simulink model "prova_LOG_raspi_09_22"  (R2020b)
settings: Solver=ode4  StartTime=0.0  StopTime=Inf  FixedStep=0.02  RelTol=1e-3  EnableMultiTasking=on
PostLoadFcn:
  | , if any(exist('dsrtsu_mdlpostloadfcn', 'file') == [2, 3, 6]), try dsrtsu_mdlpostloadfcn('Execute', bdroot); catch fprintf('Error in PostLoadFcn (dsrtsu_mdlpostloadfcn) for model "%s":\n %s\n', bdroot, lasterr); end, end,
InitFcn:
  | , if any(exist('rtifpga_mdlclblib', 'file') ~= 0), rtifpga_mdlclblib('Init', bdroot); end,
undefined symbols (not defined in the file or in its folder): DiscIntNeverNeededParam
libraries: simulink_extras x10, svdutilitieslib x4, raspberrypiCommlib x2, embdlinuxlib x1
Description:
  | Standard RTI1006 template.
  | Supported MATLAB version:  R2020b.
settings Model: Tag=RTI1006  DSRTSU_INTERNAL_RTI_VER=570  DSRTSU_INTERNAL_RTI_TYPE=rti1006  RTICANMMDATA=struct('GeneralSetupData',struct('modelroot','C:\SUBTEAMS_2021_2022\SOFTWARE_copia_vecchia\AUTOPILOTA\drive1\Load_hardware\Raspberry_v2_1','generalsettings',struct('filesettings',struct('destfolder',struct('Name','RTICANMM_FILES','Check',1),'buildfolder',struct('Name','.','Check',1),'AbsDestfolder',struct('Name','C:\SUBTEAMS_2021_2022\SOFTWARE_copia_vecchia\AUTOPILOTA\drive1\Load_hardware\Raspberry_v2_1\RTICANMM_FILES'),'AbsBuildfolder',struct('Name','C:\SUBTEAMS_2021_2022\SOFTWARE_copia_vecchia\AUTOPILOTA\drive1\Load_hardware\Raspberry_v2_1'))),'options',struct('addpaths',1,'rmpaths',1,'addtrcexclusion',true,'cannavigator',struct('checkmonitoring',0),'show_usrtrc',0,'use_usrtrc',0),'advanced',struct('options',ones(1,100)),'MPSetup',{{}},'RTI',struct('Type','ERT','Ver','','Date',''),'modelname','prova_LOG_raspi_09_22','block','prova_LOG_raspi_09_22'))  DSRTSU_INTERNAL_RTIFPGA=170  Creator=lapis-dspace  LastModifiedBy=lapis-dspace
settings SolverCC: PositivePriorityOrder=on
settings DataIOCC: SaveOutput=off  SignalLogging=off  DSMLogging=off  SaveTime=off  ReturnWorkspaceOutputs=off
settings OptimizationCC: EnhancedBackFolding=on  PassReuseOutputArgsAs=Individual arguments  MaxStackSize=64  OptimizeBlockOrder=speed  DifferentSizesBufferReuse=on  OptimizationCustomize=off  EfficientTunableParamExpr=on
settings DebuggingCC: ParameterTunabilityLossMsg=error  PregeneratedLibrarySubsystemCodeDiagnostic=none  ArithmeticOperatorsInVariantConditions=warning
settings HardwareCC: ProdBitPerPointer=32  ProdBitPerSizeT=32  ProdBitPerPtrDiffT=32  ProdLargestAtomicInteger=Long  ProdLargestAtomicFloat=Double  ProdWordSize=32  ProdLongLongMode=on  ProdHWDeviceType=ARM Compatible->ARM Cortex  TargetIntDivRoundTo=Zero  TargetEndianess=LittleEndian  TargetHWDeviceType=Custom Processor->Custom
settings ModelReferenceCC: ParallelModelReferenceMATLABWorkerInit=Load Top Model
settings SFSimCC: SimUseLocalCustomCode=off  MATLABDynamicMemAlloc=off  CustomCodeUndefinedFunction=UseInterfaceOnly
settings RTWCC: Description=Embedded Coder  SystemTargetFile=ert.tlc  HardwareBoard=Raspberry Pi  TLCOptions="-aInlineSetEventsForThisBaseRateFcn=TLC_FALSE -aSuppressMultiTaskScheduler=TLC_FALSE  -aRateBasedStepFcn=0"  TemplateMakefile=ert_default_tmf  GenerateReport=on  RTWUseLocalCustomCode=off  Toolchain=GNU GCC Raspberry Pi  BuildConfiguration=Faster Runs  IncludeHyperlinkInReport=on  LaunchReport=on  GenerateTraceInfo=on  GenerateTraceReport=on  GenerateTraceReportSl=on  GenerateTraceReportSf=on  GenerateTraceReportEml=on
settings CodeAppCC: ForceParamTrailComments=on  IgnoreCustomStorageClasses=off  OperatorAnnotations=on  SimulinkDataObjDesc=on  SFDataObjDesc=on  InsertBlockDesc=on
settings ERTTargetCC: MatFileLogging=on  SupportVariableSizeSignals=on
settings ConfigComp: CovMetricSettings=dswe

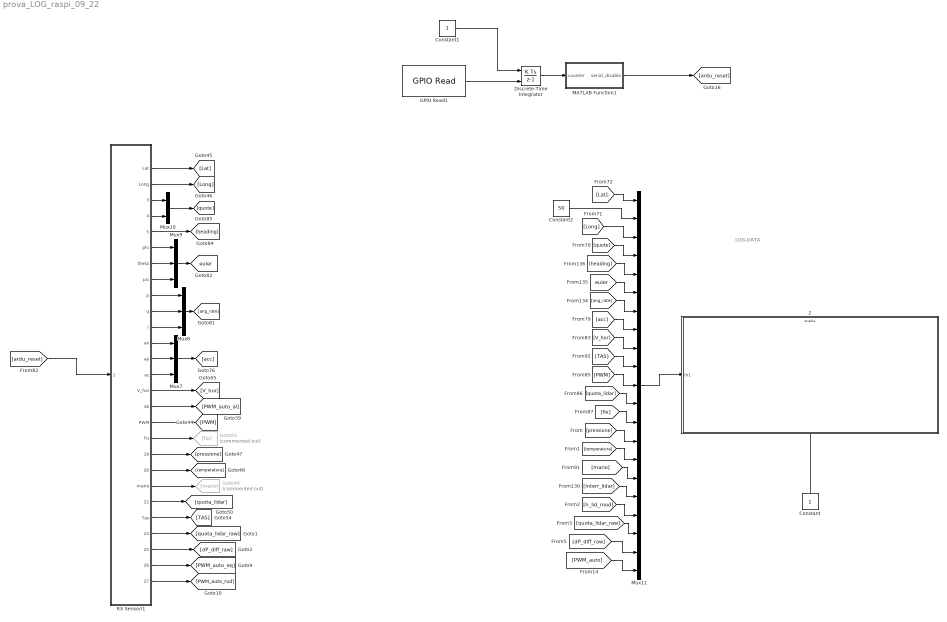
== system prova_LOG_raspi_09_22 ==
  note: LOG-DATA
  " 2" : Subsystem
  Constant : Constant
  Constant1 : Constant  SampleTime=0.02
  Constant2 : Constant  Value=50
  Discrete-Time Integrator : DiscreteIntegrator  ExternalReset=falling  SampleTime=0.02  LimitOutput=on  UpperSaturationLimit=1  LowerSaturationLimit=0  ICPrevOutput=DiscIntNeverNeededParam  ICPrevScaledInput=DiscIntNeverNeededParam
  GPIO Read1 : embdlinuxlib/GPIO Read  board=Pi 3 Model B  gpio=21  internalResistor=Off  sampleTime=0.02  direction=Input  blockPlatform=Raspberry Pi
      settings: SourceProductBaseCode=SC_BEAGLEBONE_BLUE,NVIDIA,RASPPI
  Goto49 : Goto  Commented=on  GotoTag=mario
  Goto83 : Goto  Commented=on  GotoTag=fix
  MATLAB Function1 : MATLAB Function  TreatAsAtomicUnit=on
  Mux10 : Mux  Inputs=2
  Mux11 : Mux  Inputs=21
  Mux7 : Mux  Inputs=3
  Mux8 : Mux  Inputs=3
  Mux9 : Mux  Inputs=3
  RX Sensori1 : Subsystem
  tag scope: euler=global
  wires:
  RX Sensori1/23(Tas) -> [TAS]
  RX Sensori1/10(q) -> Mux8/2
  RX Sensori1/13(ay) -> Mux7/2
  RX Sensori1/26(PWM_auto_eq) -> [PWM_auto_eq]
  RX Sensori1/4(quota_baro) -> Mux10/2
  RX Sensori1/27(PWM_auto_rud) -> [PWM_auto_rud]
  RX Sensori1/12(ax) -> Mux7/1
  RX Sensori1/14(az) -> Mux7/3
  Mux9/1 -> [euler]
  RX Sensori1/18(fix) -> Goto83/1
  RX Sensori1/25(dP_diff_raw) -> [dP_diff_raw]
  RX Sensori1/24(quota_lidar_raw) -> [quota_lidar_raw]
  RX Sensori1/15(V_hor) -> [V_hor]
  Mux8/1 -> [ang_rate]
  RX Sensori1/7(theta) -> Mux9/2
  RX Sensori1/20(temperatura) -> [temperatura]
  [ardu_reset] -> RX Sensori1/1(ardu_reset)
  RX Sensori1/5(heading) -> [heading]
  RX Sensori1/9(p) -> Mux8/1
  RX Sensori1/1(Lat) -> [Lat]
  RX Sensori1/3(quota_GPS) -> Mux10/1
  RX Sensori1/11(r) -> Mux8/3
  RX Sensori1/21(mario) -> Goto49/1
  RX Sensori1/19(pressione) -> [pressione]
  RX Sensori1/22(quota_lidar) -> [quota_lidar]
  RX Sensori1/8(psi) -> Mux9/3
  Mux10/1 -> [quote]
  RX Sensori1/16(PWM_auto_al) -> [PWM_auto_al]
  Mux7/1 -> [acc]
  RX Sensori1/2(Long) -> [Long]
  RX Sensori1/17(PWM) -> [PWM]
  RX Sensori1/6(phi) -> Mux9/1
  [acc] -> Mux11/8
  [quota_lidar_raw] -> Mux11/19
  [PWM_auto] -> Mux11/21
  [PWM] -> Mux11/11
  [dP_diff_raw] -> Mux11/20
  [h_lid_mod] -> Mux11/18
  [temperatura] -> Mux11/15
  [pressione] -> Mux11/14
  [heading] -> Mux11/5
  [Long] -> Mux11/3
  Mux11/1 -> " 2"/1(In1)
  [euler] -> Mux11/6
  [ang_rate] -> Mux11/7
  [fix] -> Mux11/13
  [Lat] -> Mux11/1
  [mario] -> Mux11/16
  [TAS] -> Mux11/10
  [quota_lidar] -> Mux11/12
  [interr_lidar] -> Mux11/17
  [quote] -> Mux11/4
  [V_hor] -> Mux11/9
  Constant/1 -> " 2"/Enable
  GPIO Read1/1 -> Discrete-Time Integrator/2
  Discrete-Time Integrator/1 -> MATLAB Function1/1(counter)
  MATLAB Function1/1(serial_disable) -> [ardu_reset]
  Constant1/1 -> Discrete-Time Integrator/1
  Constant2/1 -> Mux11/2

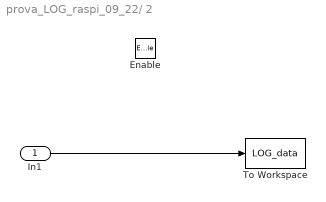
== system prova_LOG_raspi_09_22/ 2 ==
  In1 : Inport
  Enable : EnablePort
  To Workspace : ToWorkspace  VariableName=LOG_data  SaveFormat=Structure With Time  SampleTime=0.02
  wires:
  In1/1 -> To Workspace/1

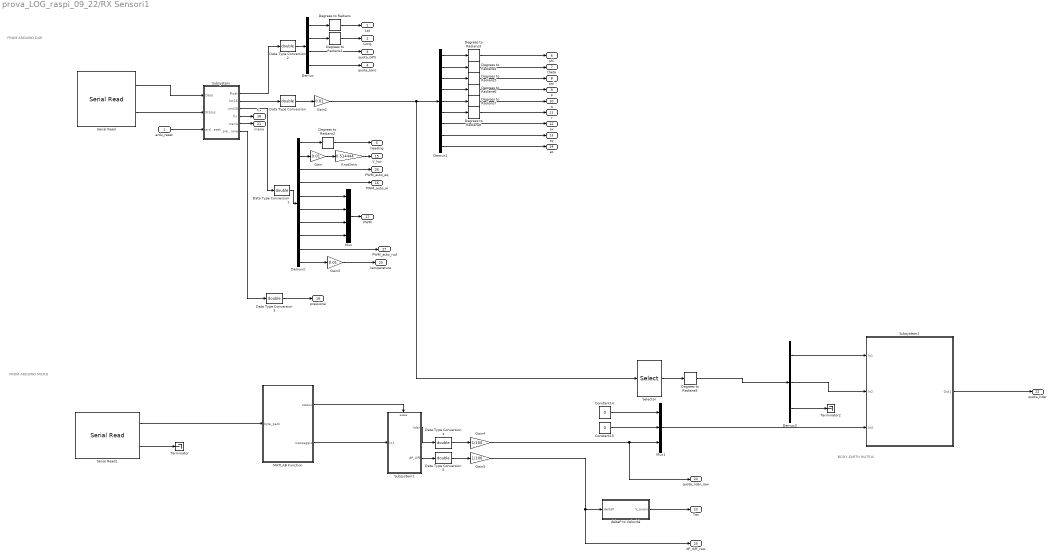
== system prova_LOG_raspi_09_22/RX Sensori1 ==
  note: FROM ARDUINO DUE
  note: FROM ARDUINO MICRO
  note: BODY-EARTH MATRIX
  ardu_reset : Inport
  Constant14 : Constant  Value=0
  Constant15 : Constant  Value=0
  Data Type Conversion{,1..5} (6 alike) : DataTypeConversion  OutDataTypeStr=double
  Degrees to Radians{,1..9} (10 alike) : simulink_extras/Transformations/Degrees to Radians
  Demux : Demux
  Demux1 : Demux  Outputs=9
  Demux2 : Demux  Outputs=10
  Demux3 : Demux  Outputs=3
  Gain : Gain  Gain=0.01
  Gain2 : Gain  Gain=0.01
  Gain3 : Gain  Gain=0.01
  Gain4 : Gain  Gain=1/100
  Gain5 : Gain  Gain=1/100
  Knot2m/s : Gain  Gain=0.514444
  MATLAB Function : MATLAB Function  TreatAsAtomicUnit=on
  Mux : Mux
  Mux1 : Mux  Inputs=3
  Selector : Selector  InputPortWidth=9  IndexOptions=Index vector (dialog)  Indices=[1:3]  OutputSizes=1
  Serial Read : raspberrypiCommlib/Serial Read  board=Pi 3 Model B+  SCIModule_=/dev/ttyACM0  Baudrate_=57600  Parity=None  StopBits_=1  HardwareFlowControl=None  ByteOrder=LittleEndian  DataLength=63  DataType=uint8  OutputStatus=on  SampleTime=0.02  blockPlatform=RaspberryPi
      settings: SourceProductBaseCode=RASPPI
  Serial Read1 : raspberrypiCommlib/Serial Read  board=Pi 3 Model B  SCIModule_=/dev/ttyACM0  Baudrate_=57600  Parity=None  StopBits_=1  HardwareFlowControl=None  ByteOrder=LittleEndian  DataLength=8  DataType=uint8  OutputStatus=on  SampleTime=0.02  blockPlatform=RaspberryPi
      settings: SourceProductBaseCode=RASPPI
  Subsystem : Subsystem
  Subsystem1 : Subsystem
  Subsystem2 : Subsystem
  Terminator : Terminator
  Terminator2 : Terminator
  deltaP to Velocità : MATLAB Function  TreatAsAtomicUnit=on
  Lat : Outport  VectorParamsAs1DForOutWhenUnconnected=off
  Long : Outport  Port=2  VectorParamsAs1DForOutWhenUnconnected=off
  quota_GPS : Outport  Port=3  VectorParamsAs1DForOutWhenUnconnected=off
  quota_baro : Outport  Port=4  VectorParamsAs1DForOutWhenUnconnected=off
  heading : Outport  Port=5  VectorParamsAs1DForOutWhenUnconnected=off
  phi : Outport  Port=6  VectorParamsAs1DForOutWhenUnconnected=off
  theta : Outport  Port=7  VectorParamsAs1DForOutWhenUnconnected=off
  psi : Outport  Port=8  VectorParamsAs1DForOutWhenUnconnected=off
  p : Outport  Port=9  VectorParamsAs1DForOutWhenUnconnected=off
  q : Outport  Port=10  VectorParamsAs1DForOutWhenUnconnected=off
  r : Outport  Port=11  VectorParamsAs1DForOutWhenUnconnected=off
  ax : Outport  Port=12  VectorParamsAs1DForOutWhenUnconnected=off
  ay : Outport  Port=13  VectorParamsAs1DForOutWhenUnconnected=off
  az : Outport  Port=14  VectorParamsAs1DForOutWhenUnconnected=off
  V_hor : Outport  Port=15  VectorParamsAs1DForOutWhenUnconnected=off
  PWM_auto_al : Outport  Port=16  VectorParamsAs1DForOutWhenUnconnected=off
  PWM : Outport  Port=17  VectorParamsAs1DForOutWhenUnconnected=off
  fix : Outport  Port=18  VectorParamsAs1DForOutWhenUnconnected=off
  pressione : Outport  Port=19  VectorParamsAs1DForOutWhenUnconnected=off
  temperatura : Outport  Port=20  VectorParamsAs1DForOutWhenUnconnected=off
  mario : Outport  Port=21  OutDataTypeStr=double  VectorParamsAs1DForOutWhenUnconnected=off
  quota_lidar : Outport  Port=22  VectorParamsAs1DForOutWhenUnconnected=off
  Tas : Outport  Port=23  VectorParamsAs1DForOutWhenUnconnected=off
  quota_lidar_raw : Outport  Port=24  VectorParamsAs1DForOutWhenUnconnected=off
  dP_diff_raw : Outport  Port=25  VectorParamsAs1DForOutWhenUnconnected=off
  PWM_auto_eq : Outport  Port=26  VectorParamsAs1DForOutWhenUnconnected=off
  PWM_auto_rud : Outport  Port=27  VectorParamsAs1DForOutWhenUnconnected=off
  wires:
  Serial Read/2 -> Subsystem/2(Status)
  Serial Read/1 -> Subsystem/1(Data)
  Subsystem/1(Float) -> Data Type Conversion2/1
  Demux/1 -> Degrees to Radians/1
  Demux/2 -> Degrees to Radians1/1
  Demux/4 -> quota_baro/1
  Subsystem/2(Int16) -> Data Type Conversion/1
  Subsystem/3(uint16) -> Data Type Conversion1/1
  Gain/1 -> Knot2m/s/1
  Demux2/3 -> PWM_auto_eq/1
  Data Type Conversion/1 -> Gain2/1
  Demux2/2 -> Gain/1
  Degrees to Radians/1 -> Lat/1
  Degrees to Radians1/1 -> Long/1
  Degrees to Radians2/1 -> heading/1
  Demux2/4 -> PWM_auto_al/1
  Demux2/7 -> Mux/3
  Demux2/8 -> Mux/4
  Data Type Conversion1/1 -> Demux2/1
  Demux2/5 -> Mux/1
  Demux2/6 -> Mux/2
  Mux/1 -> PWM/1
  Demux1/9 -> az/1
  Degrees to Radians8/1 -> r/1
  Degrees to Radians7/1 -> q/1
  Degrees to Radians6/1 -> p/1
  Degrees to Radians5/1 -> psi/1
  Degrees to Radians4/1 -> theta/1
  Degrees to Radians3/1 -> phi/1
  Demux/3 -> quota_GPS/1
  Knot2m/s/1 -> V_hor/1
  Subsystem/4(fix) -> fix/1
  Demux2/1 -> Degrees to Radians2/1
  Demux1/6 -> Degrees to Radians8/1
  Demux1/5 -> Degrees to Radians7/1
  Demux1/4 -> Degrees to Radians6/1
  Demux1/3 -> Degrees to Radians5/1
  Demux1/2 -> Degrees to Radians4/1
  Demux1/1 -> Degrees to Radians3/1
  Demux1/7 -> ax/1
  Demux1/8 -> ay/1
  Demux2/9 -> PWM_auto_rud/1
  Data Type Conversion2/1 -> Demux/1
  Gain3/1 -> temperatura/1
  Demux2/10 -> Gain3/1
  Subsystem/5(mario) -> mario/1
  Subsystem/6(pressione) -> Data Type Conversion3/1
  Data Type Conversion3/1 -> pressione/1
  ardu_reset/1 -> Subsystem/3(ardu_reset)
  MATLAB Function/2(messaggio) -> Subsystem1/1(In1)
  MATLAB Function/1(status) -> Subsystem1/Enable
  Subsystem1/1(lidar) -> Data Type Conversion4/1
  Serial Read1/1 -> MATLAB Function/1(byte_pack)
  Serial Read1/2 -> Terminator/1
  Constant15/1 -> Mux1/2
  Mux1/1 -> Subsystem2/3(In4)
  Selector/1 -> Degrees to Radians9/1
  Constant14/1 -> Mux1/1
  Degrees to Radians9/1 -> Demux3/1
  Demux3/1 -> Subsystem2/1(In1)
  Gain2/1 -> Selector/1, Demux1/1
  Data Type Conversion4/1 -> Gain4/1
  Gain4/1 -> quota_lidar_raw/1, Mux1/3
  Demux3/3 -> Terminator2/1
  Demux3/2 -> Subsystem2/2(In2)
  Subsystem2/1(Out1) -> quota_lidar/1
  Subsystem1/2(dP_diff) -> Data Type Conversion5/1
  Data Type Conversion5/1 -> Gain5/1
  deltaP to Velocità/1(V_anem) -> Tas/1
  Gain5/1 -> dP_diff_raw/1, deltaP to Velocità/1(deltaP)

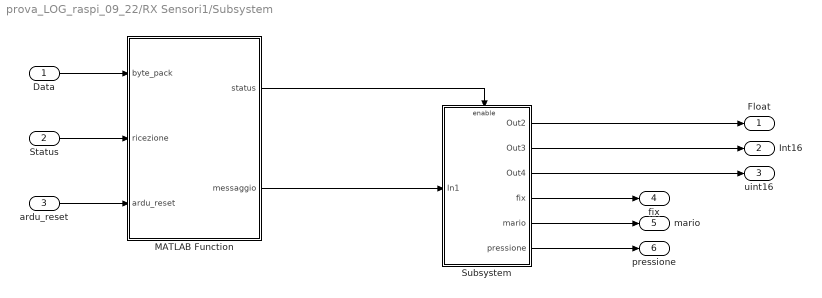
== system prova_LOG_raspi_09_22/RX Sensori1/Subsystem ==
  Data : Inport
  Status : Inport  Port=2
  ardu_reset : Inport  Port=3
  MATLAB Function : MATLAB Function  TreatAsAtomicUnit=on
  Subsystem : Subsystem
  Float : Outport  VectorParamsAs1DForOutWhenUnconnected=off
  Int16 : Outport  Port=2  VectorParamsAs1DForOutWhenUnconnected=off
  uint16 : Outport  Port=3  VectorParamsAs1DForOutWhenUnconnected=off
  fix : Outport  Port=4  VectorParamsAs1DForOutWhenUnconnected=off
  mario : Outport  Port=5  VectorParamsAs1DForOutWhenUnconnected=off
  pressione : Outport  Port=6  VectorParamsAs1DForOutWhenUnconnected=off
  wires:
  Subsystem/1(Out2) -> Float/1
  Subsystem/2(Out3) -> Int16/1
  Subsystem/3(Out4) -> uint16/1
  MATLAB Function/1(status) -> Subsystem/Enable
  MATLAB Function/2(messaggio) -> Subsystem/1(In1)
  Data/1 -> MATLAB Function/1(byte_pack)
  Status/1 -> MATLAB Function/2(ricezione)
  Subsystem/4("fix ") -> fix/1
  Subsystem/5(mario) -> mario/1
  Subsystem/6(pressione) -> pressione/1
  ardu_reset/1 -> MATLAB Function/3(ardu_reset)

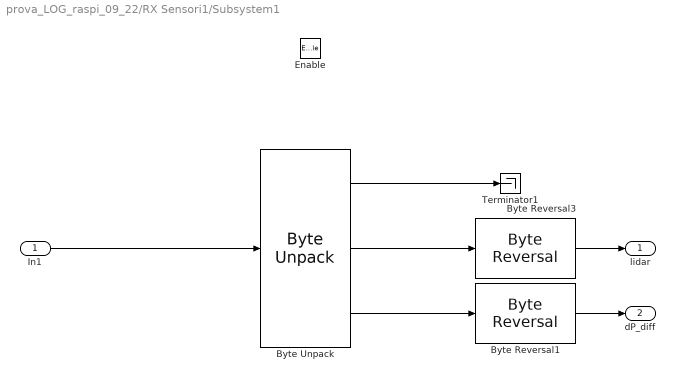
== system prova_LOG_raspi_09_22/RX Sensori1/Subsystem1 ==
  In1 : Inport
  Enable : EnablePort
  Byte Reversal1 : svdutilitieslib/Byte Reversal  numInp=1  blockPlatform=arduinoert
      settings: SourceProductBaseCode=ANDROID,ARDUINO,ML_ARDUINO,ECCORTEXA,ECCORTEXR,SC_BEAGLEBONE_BLUE,EC_FREEDOM_BOARD,EC_FRDM_K64F,INTEL_BLOCKSET,JETSONCPU,MICROBIT,NUCLEO,NVIDIA,PX4AUTOPILOTS,RASPPIIO,STMICRODIS,TIC2000,XILINX_BLOCKSET
  Byte Reversal3 : svdutilitieslib/Byte Reversal  numInp=1  blockPlatform=arduinoert
      settings: SourceProductBaseCode=ANDROID,ARDUINO,ML_ARDUINO,ECCORTEXA,ECCORTEXR,SC_BEAGLEBONE_BLUE,EC_FREEDOM_BOARD,EC_FRDM_K64F,INTEL_BLOCKSET,JETSONCPU,MICROBIT,NUCLEO,NVIDIA,PX4AUTOPILOTS,RASPPIIO,STMICRODIS,TIC2000,XILINX_BLOCKSET
  Byte Unpack : svdutilitieslib/Byte Unpack  dimensions={[2],[1],[1]}  datatypes={'uint8','uint16','int32'}  byteAlign=1  blockPlatform=arduinoert
      settings: SourceProductBaseCode=ANDROID,ARDUINO,ML_ARDUINO,ECCORTEXA,ECCORTEXR,SC_BEAGLEBONE_BLUE,EC_FREEDOM_BOARD,EC_FRDM_K64F,INTEL_BLOCKSET,JETSONCPU,MICROBIT,NUCLEO,NVIDIA,PX4AUTOPILOTS,RASPPIIO,STMICRODIS,TIC2000,XILINX_BLOCKSET
  Terminator1 : Terminator
  lidar : Outport  VectorParamsAs1DForOutWhenUnconnected=off
  dP_diff : Outport  Port=2  VectorParamsAs1DForOutWhenUnconnected=off
  wires:
  In1/1 -> Byte Unpack/1
  Byte Unpack/1 -> Terminator1/1
  Byte Unpack/2 -> Byte Reversal3/1
  Byte Reversal3/1 -> lidar/1
  Byte Unpack/3 -> Byte Reversal1/1
  Byte Reversal1/1 -> dP_diff/1

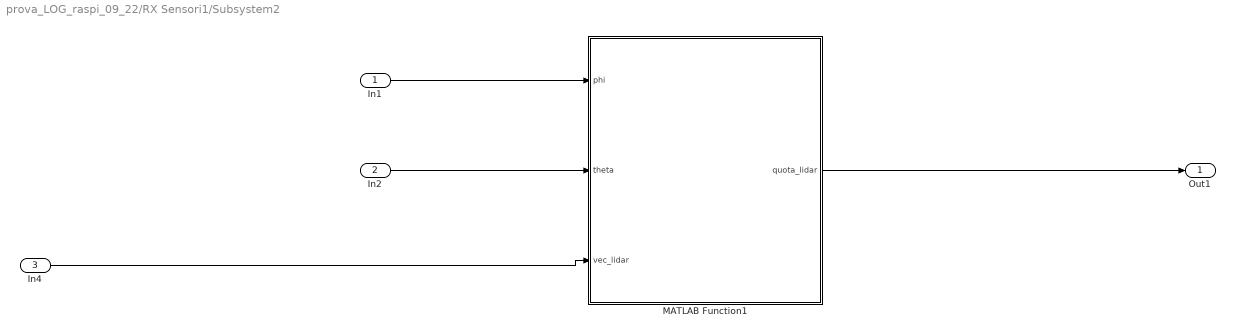
== system prova_LOG_raspi_09_22/RX Sensori1/Subsystem2 ==
  In1 : Inport
  In2 : Inport  Port=2
  In4 : Inport  Port=3
  MATLAB Function1 : MATLAB Function  TreatAsAtomicUnit=on
  Out1 : Outport  VectorParamsAs1DForOutWhenUnconnected=off
  wires:
  In4/1 -> MATLAB Function1/3(vec_lidar)
  MATLAB Function1/1(quota_lidar) -> Out1/1
  In1/1 -> MATLAB Function1/1(phi)
  In2/1 -> MATLAB Function1/2(theta)

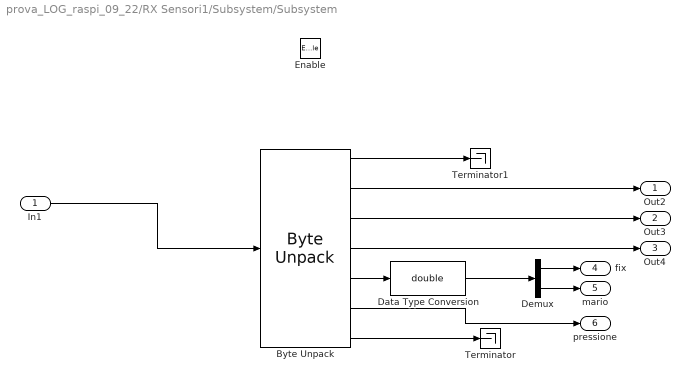
== system prova_LOG_raspi_09_22/RX Sensori1/Subsystem/Subsystem ==
  In1 : Inport
  Enable : EnablePort
  Byte Unpack : svdutilitieslib/Byte Unpack  dimensions={[2],[4],[9],[10],[2],[1],[1]}  datatypes={'uint8','single','int16','uint16','uint8','uint32','uint8'}  byteAlign=1  blockPlatform=arduinoert
      settings: SourceProductBaseCode=ANDROID,ARDUINO,ML_ARDUINO,ECCORTEXA,ECCORTEXR,SC_BEAGLEBONE_BLUE,EC_FREEDOM_BOARD,EC_FRDM_K64F,INTEL_BLOCKSET,JETSONCPU,MICROBIT,NUCLEO,NVIDIA,PX4AUTOPILOTS,RASPPIIO,STMICRODIS,TIC2000,XILINX_BLOCKSET
  Data Type Conversion : DataTypeConversion  OutDataTypeStr=double
  Demux : Demux  Outputs=2
  Terminator : Terminator
  Terminator1 : Terminator
  Out2 : Outport  VectorParamsAs1DForOutWhenUnconnected=off
  Out3 : Outport  Port=2  VectorParamsAs1DForOutWhenUnconnected=off
  Out4 : Outport  Port=3  VectorParamsAs1DForOutWhenUnconnected=off
  "fix " : Outport  Port=4  VectorParamsAs1DForOutWhenUnconnected=off
  mario : Outport  Port=5  VectorParamsAs1DForOutWhenUnconnected=off
  pressione : Outport  Port=6  VectorParamsAs1DForOutWhenUnconnected=off
  wires:
  In1/1 -> Byte Unpack/1
  Byte Unpack/1 -> Terminator1/1
  Byte Unpack/4 -> Out4/1
  Byte Unpack/3 -> Out3/1
  Byte Unpack/2 -> Out2/1
  Byte Unpack/7 -> Terminator/1
  Byte Unpack/5 -> Data Type Conversion/1
  Demux/1 -> "fix "/1
  Demux/2 -> mario/1
  Data Type Conversion/1 -> Demux/1
  Byte Unpack/6 -> pressione/1

== matlab function prova_LOG_raspi_09_22/MATLAB Function1 ==
  data: counter input; serial_disable output
function serial_disable = fcn(counter)

if counter < 1
    serial_disable = 0;
else
    serial_disable = 1;
end

== matlab function prova_LOG_raspi_09_22/RX Sensori1/deltaP to Velocità ==
  data: deltaP input; V_anem output
function V_anem = fcn(deltaP)


rho_0=1.225;
V_anem=sqrt(2*abs(deltaP)/rho_0);

== matlab function prova_LOG_raspi_09_22/RX Sensori1/MATLAB Function ==
  data: byte_pack input; status output; messaggio output
function [status,messaggio]  = LETTURA_Arduino_mex(byte_pack)



status = false;                                        %ho aggiunto questo
messaggio = uint8(zeros(1,8)) ;
M = uint8(length(byte_pack)) ;

 





    for i = 1 : M-1  
        if ( byte_pack(i) == 254 &&  byte_pack(i + 1) == 255 )                  % mi conviene mandare un secondo byte all'inizio cosi non devo cambiare nulla
            messaggio(1:end) = byte_pack(i:i+7) ;
            status = true ; 
            break
        end
    end   % lho messo qua

== matlab function prova_LOG_raspi_09_22/RX Sensori1/Subsystem/MATLAB Function ==
  data: byte_pack input; status output; messaggio output; ricezione input; ardu_reset input
function [status,messaggio]  = LETTURA_Arduino_mex(byte_pack,ricezione,ardu_reset)

persistent message counter start_found

status = false;                                        %ho aggiunto questo
messaggio = uint8(zeros(1,63)) ;
M = uint8(length(byte_pack)) ;
entrata = true ;

if isempty(start_found) 
     start_found = false ;
end 
if isempty (counter) 
    counter = uint8(0) ;
end 
if isempty(message)
     message = uint8(zeros(1,63)) ;
end

if ((ricezione ~= 0) || (ardu_reset == 0))
    start_found = false ;
    message = uint8(zeros(1,63)) ;
    counter = uint8(0)  ;
    entrata = false ;
end

if (start_found == 0 && entrata == true )
    for i = 1 : M-1  
        if ( byte_pack(i) == 62 &&  byte_pack(i + 1) == 255 )                  % mi conviene mandare un secondo byte all'inizio cosi non devo cambiare nulla
            message(1:M - (i-1)) = byte_pack(i:end) ;
            counter = M - (i-1) ; 
            start_found = true ;
            break
        end
    end   % lho messo qua
        if counter == M 
            messaggio = message ;
            message = uint8(zeros(1,63)) ;
            status = true ;
            start_found = false ;
            counter = uint8(0) ;
        end
     %end
    
    
elseif start_found == 1 

        message(counter + 1 : end) = byte_pack(1:M - counter) ;
        status = true;       %ho aggiunto questo
        messaggio = message ;
        counter = M - counter ;
        message = uint8(zeros(1,63)) ;
        
            for i = counter : M-1  
        if ( byte_pack(i) == 62 &&  byte_pack(i + 1) == 255 )                  % mi conviene mandare un secondo byte all'inizio cosi non devo cambiare nulla
            message(1:M - (i-1)) = byte_pack(i:end) ;
            counter = M - (i-1) ; 
            start_found = true ;
            break
        else 
            start_found = false ;
            counter = uint8(0);
        end 
            end
        
     %   message (1 : M-counter ) = byte_pack(counter + 1:end) ;
     %   counter = M - counter ;

end

== matlab function prova_LOG_raspi_09_22/RX Sensori1/Subsystem2/MATLAB Function1 ==
  data: phi input; quota_lidar output; theta input; vec_lidar input
function quota_lidar = fcn(phi,theta,vec_lidar)

vec_quota = [0; 0; 0];


LBE = [cos(theta)           sin(phi)*sin(theta)       cos(phi)*sin(theta);
       0                       cos(phi)                  -sin(phi);
       -sin(theta)          cos(theta)*sin(phi)       cos(phi)*cos(theta)];
       

vec_quota = LBE*vec_lidar;   % componenti della quota lidar in assi NED

quota_lidar = vec_quota(3);     % prendo la componente Z perchè mi interessa la quota
